simulink model "main"  (R2022a)
settings: Solver=FixedStepDiscrete  StartTime=0.0  StopTime=Inf  FixedStep=(50e-6)-(sim_en*4.995e-5)  RelTol=1e-3  EnableMultiTasking=on
model workspace (MAT data in the model file):
  Param : Simulink.Parameter (value not decoded)
  ac_ok : Simulink.Signal (value not decoded)
  ac_ok_120 : Simulink.Signal (value not decoded)
  bulk_voltage : Simulink.Signal (value not decoded)
  burstduty_integ_max : Simulink.Signal (value not decoded)
  burstduty_integ_min : Simulink.Signal (value not decoded)
  burstduty_ki : Simulink.Signal (value not decoded)
  burstduty_kp : Simulink.Signal (value not decoded)
  calib_ok : Simulink.Signal (value not decoded)
  can_addr1 : Simulink.Signal (value not decoded)
  can_addr2 : Simulink.Signal (value not decoded)
  can_addr3 : Simulink.Signal (value not decoded)
  can_addr4 : Simulink.Signal (value not decoded)
  can_data_rx : Simulink.Signal (value not decoded)
  can_data_tx : Simulink.Signal (value not decoded)
  can_timeout_120 : Simulink.Signal (value not decoded)
  chksum_scircv : Simulink.Signal (value not decoded)
  clllc_en_120 : Simulink.Signal (value not decoded)
  clllc_fault_120 : Simulink.Signal (value not decoded)
  clllc_ok_120 : Simulink.Signal (value not decoded)
  cmpss1h : Simulink.Signal (value not decoded)
  cmpss1l : Simulink.Signal (value not decoded)
  cmpss2h : Simulink.Signal (value not decoded)
  cmpss2l : Simulink.Signal (value not decoded)
  cmpss3h : Simulink.Signal (value not decoded)
  cmpss3l : Simulink.Signal (value not decoded)
  cmpss4h : Simulink.Signal (value not decoded)
  cmpss4l : Simulink.Signal (value not decoded)
  cmpss5h : Simulink.Signal (value not decoded)
  cmpss5l : Simulink.Signal (value not decoded)
  cmpss6h : Simulink.Signal (value not decoded)
  cmpss6l : Simulink.Signal (value not decoded)
  cmpss7h : Simulink.Signal (value not decoded)
  cmpss7l : Simulink.Signal (value not decoded)
  cmpss8h : Simulink.Signal (value not decoded)
  cmpss8l : Simulink.Signal (value not decoded)
  cnt_idle : Simulink.Signal (value not decoded)
  cnt_orps : Simulink.Signal (value not decoded)
  cnt_scircv : Simulink.Signal (value not decoded)
  cnt_scixmt : Simulink.Signal (value not decoded)
  cnt_scixmt_func : Simulink.Signal (value not decoded)
  cnt_temp_mux : Simulink.Signal (value not decoded)
  cnt_vdroop : Simulink.Signal (value not decoded)
  config_ok : Simulink.Signal (value not decoded)
  control_en : Simulink.Signal (value not decoded)
  cp_ready_120 : Simulink.Signal (value not decoded)
  d2d_en : Simulink.Signal (value not decoded)
  dchg_off : Simulink.Signal (value not decoded)
  debug_dacb : Simulink.Signal (value not decoded)
  debug_dacc : Simulink.Signal (value not decoded)
  debug_msg1 : Simulink.Signal (value not decoded)
  debug_msg2 : Simulink.Signal (value not decoded)
  debug_msg3 : Simulink.Signal (value not decoded)
  debug_msg4 : Simulink.Signal (value not decoded)
  debug_msg5 : Simulink.Signal (value not decoded)
  debug_msg6 : Simulink.Signal (value not decoded)
  dir_v2g : Simulink.Signal (value not decoded)
  eoss_llc1 : Simulink.Signal (value not decoded)
  eoss_llc2 : Simulink.Signal (value not decoded)
  eoss_orps : Simulink.Signal (value not decoded)
  fault_ocp : Simulink.Signal (value not decoded)
  fault_otp : Simulink.Signal (value not decoded)
  fault_ovp : Simulink.Signal (value not decoded)
  fut_en : Simulink.Signal (value not decoded)
  fwd_en_120 : Simulink.Signal (value not decoded)
  gain_llc1_sec_idc : Simulink.Signal (value not decoded)
  gain_llc1_temp_sr : Simulink.Signal (value not decoded)
  gain_llc2_sec_idc : Simulink.Signal (value not decoded)
  gain_vbat : Simulink.Signal (value not decoded)
  gain_vbulk : Simulink.Signal (value not decoded)
  gain_vout : Simulink.Signal (value not decoded)
  input_current_phasea : Simulink.Signal (value not decoded)
  input_current_phaseb : Simulink.Signal (value not decoded)
  input_current_phasec : Simulink.Signal (value not decoded)
  input_freq : Simulink.Signal (value not decoded)
  input_power : Simulink.Signal (value not decoded)
  input_voltage_phasea : Simulink.Signal (value not decoded)
  input_voltage_phaseb : Simulink.Signal (value not decoded)
  input_voltage_phasec : Simulink.Signal (value not decoded)
  ishare_arbiter : Simulink.Signal (value not decoded)
  ishare_thresh : Simulink.Signal (value not decoded)
  led_g : Simulink.Signal (value not decoded)
  led_r : Simulink.Signal (value not decoded)
  led_y : Simulink.Signal (value not decoded)
  llc1_burst_integ : Simulink.Signal (value not decoded)
  llc1_burstduty_buffer : Simulink.Signal (value not decoded)
  llc1_pfm_error : Simulink.Signal (value not decoded)
  llc1_pfm_integ : Simulink.Signal (value not decoded)
  llc1_pfm_prop : Simulink.Signal (value not decoded)
  llc1_pri_idc : Simulink.Signal (value not decoded)
  llc1_ps_buffer : Simulink.Signal (value not decoded)
  llc1_pspwm_error : Simulink.Signal (value not decoded)
  llc1_pspwm_integ : Simulink.Signal (value not decoded)
  llc1_pspwm_prop : Simulink.Signal (value not decoded)
  llc1_sec_idc : Simulink.Signal (value not decoded)
  llc1_temp_sr : Simulink.Signal (value not decoded)
  llc1_ts_tbctr_buffer : Simulink.Signal (value not decoded)
  llc2_burst_integ : Simulink.Signal (value not decoded)
  llc2_burstduty_buffer : Simulink.Signal (value not decoded)
  llc2_en : Simulink.Signal (value not decoded)
  llc2_en_buffer : Simulink.Signal (value not decoded)
  llc2_pfm_error : Simulink.Signal (value not decoded)
  llc2_pfm_integ : Simulink.Signal (value not decoded)
  llc2_pfm_prop : Simulink.Signal (value not decoded)
  llc2_pri_idc : Simulink.Signal (value not decoded)
  llc2_ps_buffer : Simulink.Signal (value not decoded)
  llc2_pspwm_error : Simulink.Signal (value not decoded)
  llc2_pspwm_integ : Simulink.Signal (value not decoded)
  llc2_pspwm_prop : Simulink.Signal (value not decoded)
  llc2_sec_idc : Simulink.Signal (value not decoded)
  llc2_temp_sr : Simulink.Signal (value not decoded)
  llc2_ts_tbctr_buffer : Simulink.Signal (value not decoded)
  loop_adcint : Simulink.Signal (value not decoded)
  loop_control : Simulink.Signal (value not decoded)
  loop_idle : Simulink.Signal (value not decoded)
  mid_bulk_voltage : Simulink.Signal (value not decoded)
  mode_120 : Simulink.Signal (value not decoded)
  mode_cc_cv : Simulink.Signal (value not decoded)
  myParam : mpt.Parameter (value not decoded)
  obc_ok_120 : Simulink.Signal (value not decoded)
  offset_llc1_sec_idc : Simulink.Signal (value not decoded)
  offset_llc1_temp_sr : Simulink.Signal (value not decoded)
  offset_llc2_sec_idc : Simulink.Signal (value not decoded)
  offset_vbat : Simulink.Signal (value not decoded)
  offset_vbulk : Simulink.Signal (value not decoded)
  offset_vout : Simulink.Signal (value not decoded)
  openloop_en : Simulink.Signal (value not decoded)
  openloop_fault_en : Simulink.Signal (value not decoded)
  ot_fault_120 : Simulink.Signal (value not decoded)
  pfc_en : Simulink.Signal (value not decoded)
  pfc_en_120 : Simulink.Signal (value not decoded)
  pfc_fw_revision : Simulink.Signal (value not decoded)
  pfc_fw_revision_bootloader : Simulink.Signal (value not decoded)
  pfc_fw_revision_debug : Simulink.Signal (value not decoded)
  pfc_ok : Simulink.Signal (value not decoded)
  pfc_ok_120 : Simulink.Signal (value not decoded)
  pfm_a0 : Simulink.Signal (value not decoded)
  pfm_a1 : Simulink.Signal (value not decoded)
  pfm_integ_max : Simulink.Signal (value not decoded)
  pfm_integ_min : Simulink.Signal (value not decoded)
  pfm_ki : Simulink.Signal (value not decoded)
  pfm_kp : Simulink.Signal (value not decoded)
  pri_fut_en : Simulink.Signal (value not decoded)
  pri_fut_en_buffer : Simulink.Signal (value not decoded)
  pri_halfbridge_en : Simulink.Signal (value not decoded)
  pri_halfbridge_en_buffer : Simulink.Signal (value not decoded)
  pspwm_integ_max : Simulink.Signal (value not decoded)
  pspwm_integ_min : Simulink.Signal (value not decoded)
  pspwm_ki : Simulink.Signal (value not decoded)
  pspwm_kp : Simulink.Signal (value not decoded)
  ref_idclink_max : Simulink.Signal (value not decoded)
  ref_iout : Simulink.Signal (value not decoded)
  ref_iout_calib : Simulink.Signal (value not decoded)
  ref_iout_llc1 : Simulink.Signal (value not decoded)
  ref_iout_llc1_calib : Simulink.Signal (value not decoded)
  ref_iout_llc2 : Simulink.Signal (value not decoded)
  ref_iout_llc2_calib : Simulink.Signal (value not decoded)
  ref_pout : Simulink.Signal (value not decoded)
  ref_ss_llc1 : Simulink.Signal (value not decoded)
  ref_ss_llc2 : Simulink.Signal (value not decoded)
  ref_ss_orps : Simulink.Signal (value not decoded)
  ref_vbat : Simulink.Signal (value not decoded)
  ref_vbat_calib : Simulink.Signal (value not decoded)
  ref_vbulk : Simulink.Signal (value not decoded)
  ref_vbulk_calib : Simulink.Signal (value not decoded)
  ref_vbulk_llc1_calib : Simulink.Signal (value not decoded)
  ref_vbulk_llc2_calib : Simulink.Signal (value not decoded)
  ref_vout : Simulink.Signal (value not decoded)
  ref_vout_calib : Simulink.Signal (value not decoded)
  relay_en : Simulink.Signal (value not decoded)
  reset_flag : Simulink.Signal (value not decoded)
  rev_en_120 : Simulink.Signal (value not decoded)
  runtime_control : Simulink.Signal (value not decoded)
  runtime_idle : Simulink.Signal (value not decoded)
  scircv_buffer : Simulink.Signal (value not decoded)
  scircv_buffer_tmp : Simulink.Signal (value not decoded)
  scircv_buffer_tmp_idx0 : Simulink.Signal (value not decoded)
  scircv_chksum : Simulink.Signal (value not decoded)
  scircv_chksum_ok : Simulink.Signal (value not decoded)
  scircv_parse_ok : Simulink.Signal (value not decoded)
  scixmt_buffer : Simulink.Signal (value not decoded)
  scixmt_chksum : Simulink.Signal (value not decoded)
  scixmt_func : Simulink.Signal (value not decoded)
  scixmt_word0_lsb : Simulink.Signal (value not decoded)
  scixmt_word0_msb : Simulink.Signal (value not decoded)
  scixmt_word1_lsb : Simulink.Signal (value not decoded)
  scixmt_word1_msb : Simulink.Signal (value not decoded)
  scixmt_word2_lsb : Simulink.Signal (value not decoded)
  scixmt_word2_msb : Simulink.Signal (value not decoded)
  scixmt_wr : Simulink.Signal (value not decoded)
  ss_step : Simulink.Signal (value not decoded)
  state_calib : Simulink.Signal (value not decoded)
  state_control : Simulink.Signal (value not decoded)
  state_hkeep : Simulink.Signal (value not decoded)
  status_cmpss : Simulink.Signal (value not decoded)
  status_control : Simulink.Signal (value not decoded)
  status_digin : Simulink.Signal (value not decoded)
  status_digout : Simulink.Signal (value not decoded)
  status_fault : Simulink.Signal (value not decoded)
  status_input : Simulink.Signal (value not decoded)
  status_pfc : Simulink.Signal (value not decoded)
  temp_inlet : Simulink.Signal (value not decoded)
  temp_llc1_fet_hs : Simulink.Signal (value not decoded)
  temp_llc2_fet_hs : Simulink.Signal (value not decoded)
  temp_mux : Simulink.Signal (value not decoded)
  temp_mux_s0 : Simulink.Signal (value not decoded)
  temp_mux_s1 : Simulink.Signal (value not decoded)
  temp_mux_s2 : Simulink.Signal (value not decoded)
  temp_outlet : Simulink.Signal (value not decoded)
  temp_pfc_fet_hsa : Simulink.Signal (value not decoded)
  temp_pfc_fet_hsb : Simulink.Signal (value not decoded)
  temp_pfc_fet_hsc : Simulink.Signal (value not decoded)
  temp_pfc_fet_lsa : Simulink.Signal (value not decoded)
  temp_pfc_fet_lsb : Simulink.Signal (value not decoded)
  temp_pfc_fet_lsc : Simulink.Signal (value not decoded)
  test_mode : Simulink.Signal (value not decoded)
  tfcv_cc : Simulink.Signal (value not decoded)
  tfcv_cc_llc2 : Simulink.Signal (value not decoded)
  tfcv_cv : Simulink.Signal (value not decoded)
  tfcv_sr_en : Simulink.Signal (value not decoded)
  tfv_assert_llc1_pri_idc : Simulink.Signal (value not decoded)
  tfv_assert_llc1_sec_idc : Simulink.Signal (value not decoded)
  tfv_assert_llc1_temp_sr : Simulink.Signal (value not decoded)
  tfv_assert_llc2_pri_idc : Simulink.Signal (value not decoded)
  tfv_assert_llc2_sec_idc : Simulink.Signal (value not decoded)
  tfv_assert_llc2_temp_sr : Simulink.Signal (value not decoded)
  tfv_assert_temp_outlet : Simulink.Signal (value not decoded)
  tfv_assert_vaux_uv : Simulink.Signal (value not decoded)
  tfv_assert_vbat : Simulink.Signal (value not decoded)
  tfv_assert_vbulk : Simulink.Signal (value not decoded)
  tfv_assert_vout : Simulink.Signal (value not decoded)
  tfv_cnt_tz : Simulink.Signal (value not decoded)
  tfv_deassert_llc1_pri_idc : Simulink.Signal (value not decoded)
  tfv_deassert_llc1_sec_idc : Simulink.Signal (value not decoded)
  tfv_deassert_llc1_temp_sr : Simulink.Signal (value not decoded)
  tfv_deassert_llc2_pri_idc : Simulink.Signal (value not decoded)
  tfv_deassert_llc2_sec_idc : Simulink.Signal (value not decoded)
  tfv_deassert_llc2_temp_sr : Simulink.Signal (value not decoded)
  tfv_deassert_temp_outlet : Simulink.Signal (value not decoded)
  tfv_deassert_vaux_uv : Simulink.Signal (value not decoded)
  tfv_deassert_vbat : Simulink.Signal (value not decoded)
  tfv_deassert_vbulk : Simulink.Signal (value not decoded)
  tfv_deassert_vout : Simulink.Signal (value not decoded)
  tfv_llc1_pri_idc : Simulink.Signal (value not decoded)
  tfv_llc1_sec_idc : Simulink.Signal (value not decoded)
  tfv_llc1_temp_sr : Simulink.Signal (value not decoded)
  tfv_llc2_pri_idc : Simulink.Signal (value not decoded)
  tfv_llc2_sec_idc : Simulink.Signal (value not decoded)
  tfv_llc2_temp_sr : Simulink.Signal (value not decoded)
  tfv_temp_outlet : Simulink.Signal (value not decoded)
  tfv_vaux_uv : Simulink.Signal (value not decoded)
  tfv_vbat : Simulink.Signal (value not decoded)
  tfv_vbulk : Simulink.Signal (value not decoded)
  tfv_vout : Simulink.Signal (value not decoded)
  timer_1ms : Simulink.Signal (value not decoded)
  tz : Simulink.Signal (value not decoded)
  valve_en : Simulink.Signal (value not decoded)
  vaux : Simulink.Signal (value not decoded)
  vbat : Simulink.Signal (value not decoded)
  vbulk : Simulink.Signal (value not decoded)
  vout : Simulink.Signal (value not decoded)
undefined symbols (not defined in the file or in its folder): CAN_O_INT, CANA_BASE, Down, GPTRIP1SEL, GPTRIP2SEL, TZ1, TZ2, Up
libraries: hdlsllib x159, simulink x94, c2802xlib x32, c2837xDlib x19, c2807xlib x16, c280xlib x13, canmsglib x8, idelinklib_common x2, c2000lib x1, c281xlib x1
(part 18 of 20)

== system main/Task_Manager/Tmr_20mS/codegen/Task_20mS/Tx_Handler/Run Tx Routine/TxReadRequest/Tx TxDeb Dat2 147 ==
  Action Port : ActionPort  ActionPortLabel=case [ 210 ]:
  CAN Pack1 : canmsglib/CAN Pack  MsgList=(none)  MsgName=CAN Msg  MsgIDType=Standard (11-bit identifier)  MsgIdentifier=0x147  MsgLength=8  Remote=off  ApplyMinMax=off  BusOutput=off  SignalInfo={}
      settings: SourceProductBaseCode=XP,ME,VN  DataFormat=raw data
  Constant4 : Constant  Value=0  OutDataTypeStr=uint8
  Data Store Read1 : DataStoreRead  DataStoreName=u16Debug3  IndexOptions=Index vector (dialog)  Indices=1  OutputSizes=1
  Data Store Read2 : DataStoreRead  DataStoreName=u16Debug4  IndexOptions=Index vector (dialog)  Indices=1  OutputSizes=1
  Data Store Read3 : DataStoreRead  DataStoreName=u16Debug5  IndexOptions=Index vector (dialog)  Indices=1  OutputSizes=1
  Vector Concatenate : Concatenate  NumInputs=8
  eCAN Transmit : c280xlib/eCAN Transmit  chipFamily=C280x  useModule=eCAN_A  mailboxNo=8  messageID=hex2dec('0147')  messageType=Standard (11-bit identifier)  enableBlockingMode=off  postInterrupt=off  interruptLine=0
      settings: SourceProductBaseCode=TIC2000
  u16 Data to Bytes : Subsystem
  u16 Data to Bytes1 : Subsystem
  u16 Data to Bytes2 : Subsystem
  wires:
  u16 Data to Bytes1/2(u8Msb) -> Vector Concatenate/6
  u16 Data to Bytes2/2(u8Msb) -> Vector Concatenate/4
  u16 Data to Bytes1/1(u8Lsb) -> Vector Concatenate/5
  Data Store Read1/1 -> u16 Data to Bytes/1(u16 Data)
  Data Store Read3/1 -> u16 Data to Bytes1/1(u16 Data)
  Vector Concatenate/1 -> CAN Pack1/1
  u16 Data to Bytes/1(u8Lsb) -> Vector Concatenate/1
  CAN Pack1/1 -> eCAN Transmit/1
  Data Store Read2/1 -> u16 Data to Bytes2/1(u16 Data)
  u16 Data to Bytes/2(u8Msb) -> Vector Concatenate/2
  Constant4/1 -> Vector Concatenate/8, Vector Concatenate/7
  u16 Data to Bytes2/1(u8Lsb) -> Vector Concatenate/3

== system main/Task_Manager/Tmr_20mS/codegen/Task_20mS/Tx_Handler/Run Tx Routine/TxStatusData/Tx Sec Status ID120 ==
  Action Port : ActionPort  ActionPortLabel=case [ 0 ]:
  CAN Pack1 : canmsglib/CAN Pack  MsgList=(none)  MsgName=CAN Msg  MsgIDType=Standard (11-bit identifier)  MsgIdentifier=0x120  MsgLength=8  Remote=off  ApplyMinMax=off  BusOutput=off  SignalInfo={}
      settings: SourceProductBaseCode=XP,ME,VN  DataFormat=raw data
  Constant1 : Constant  Value=0.1  OutDataTypeStr=single
  Constant3 : Constant  Value=0.01  OutDataTypeStr=single
  Constant4 : Constant  Value=0.1  OutDataTypeStr=single
  Data Store Read1 : DataStoreRead  DataStoreName=sSecStatus  IndexOptions=Index vector (dialog)  Indices=1  OutputSizes=1
  Data Store Read2 : DataStoreRead  DataStoreName=f32Vout  IndexOptions=Index vector (dialog)  Indices=1  OutputSizes=1
  Data Store Read3 : DataStoreRead  DataStoreName=b00_DebugEnabled  IndexOptions=Index vector (dialog)  Indices=1  OutputSizes=1
  Data Store Read4 : DataStoreRead  DataStoreName=f32Iout  IndexOptions=Index vector (dialog)  Indices=1  OutputSizes=1
  Data Store Read5 : DataStoreRead  DataStoreName=f32Vbulk  IndexOptions=Index vector (dialog)  Indices=1  OutputSizes=1
  Float Data to Bytes : Subsystem
  Float Data to Bytes1 : Subsystem
  Float Data to Bytes2 : Subsystem
  If1 : If  IfExpression=u1 == 1
  TxReadRequest : Subsystem  TreatAsAtomicUnit=on
  Vector Concatenate : Concatenate  NumInputs=8
  eCAN Transmit : c280xlib/eCAN Transmit  chipFamily=C280x  useModule=eCAN_A  mailboxNo=0  messageID=hex2dec('0120')  messageType=Standard (11-bit identifier)  enableBlockingMode=off  postInterrupt=off  interruptLine=0
      settings: SourceProductBaseCode=TIC2000
  u16 Data to Bytes : Subsystem
  wires:
  CAN Pack1/1 -> eCAN Transmit/1
  Data Store Read3/1 -> If1/1
  If1/1 -> TxReadRequest/Action
  Data Store Read1/1 -> u16 Data to Bytes/1(u16 Data)
  u16 Data to Bytes/1(u8Lsb) -> Vector Concatenate/1
  u16 Data to Bytes/2(u8Msb) -> Vector Concatenate/2
  Vector Concatenate/1 -> CAN Pack1/1
  Constant1/1 -> Float Data to Bytes/2(Resol.)
  Data Store Read2/1 -> Float Data to Bytes/1(Float Data)
  Float Data to Bytes/1(u8Lsb) -> Vector Concatenate/3
  Float Data to Bytes/2(u8Msb) -> Vector Concatenate/4
  Data Store Read4/1 -> Float Data to Bytes1/1(Float Data)
  Constant3/1 -> Float Data to Bytes1/2(Resol.)
  Constant4/1 -> Float Data to Bytes2/2(Resol.)
  Data Store Read5/1 -> Float Data to Bytes2/1(Float Data)
  Float Data to Bytes1/1(u8Lsb) -> Vector Concatenate/5
  Float Data to Bytes1/2(u8Msb) -> Vector Concatenate/6
  Float Data to Bytes2/1(u8Lsb) -> Vector Concatenate/7
  Float Data to Bytes2/2(u8Msb) -> Vector Concatenate/8

== system main/Task_Manager/Tmr_20mS/codegen/Task_20mS/Tx_Handler/Run Tx Routine/TxStatusData/Tx Sec1 ID140 ==
  Action Port : ActionPort  ActionPortLabel=case [ 1 ]:
  CAN Pack1 : canmsglib/CAN Pack  MsgList=(none)  MsgName=CAN Msg  MsgIDType=Standard (11-bit identifier)  MsgIdentifier=0x140  MsgLength=8  Remote=off  ApplyMinMax=off  BusOutput=off  SignalInfo={}
      settings: SourceProductBaseCode=XP,ME,VN  DataFormat=raw data
  Constant1 : Constant  Value=2  OutDataTypeStr=uint8
  Constant4 : Constant  Value=0.01  OutDataTypeStr=single
  Data Store Read1 : DataStoreRead  DataStoreName=sSecFault  IndexOptions=Index vector (dialog)  Indices=1  OutputSizes=1
  Data Store Read2 : DataStoreRead  DataStoreName=u16Reserved1  IndexOptions=Index vector (dialog)  Indices=1  OutputSizes=1
  Data Store Read3 : DataStoreRead  DataStoreName=u16Reserved2  IndexOptions=Index vector (dialog)  Indices=1  OutputSizes=1
  Data Store Read5 : DataStoreRead  DataStoreName=f32PriCurrRev  IndexOptions=Index vector (dialog)  Indices=1  OutputSizes=1
  Data Store Write1 : DataStoreWrite  DataStoreName=u8CanTxIndex  IndexOptions=Index vector (dialog)  Indices=1  OutputSizes=1
  Float Data to Bytes2 : Subsystem
  Vector Concatenate : Concatenate  NumInputs=8
  eCAN Transmit : c280xlib/eCAN Transmit  chipFamily=C280x  useModule=eCAN_A  mailboxNo=1  messageID=hex2dec('0140')  messageType=Standard (11-bit identifier)  enableBlockingMode=off  postInterrupt=off  interruptLine=0
      settings: SourceProductBaseCode=TIC2000
  u16 Data to Bytes : Subsystem
  u16 Data to Bytes1 : Subsystem
  u16 Data to Bytes2 : Subsystem
  wires:
  Constant1/1 -> Data Store Write1/1
  Data Store Read2/1 -> u16 Data to Bytes2/1(u16 Data)
  CAN Pack1/1 -> eCAN Transmit/1
  u16 Data to Bytes2/1(u8Lsb) -> Vector Concatenate/3
  u16 Data to Bytes/1(u8Lsb) -> Vector Concatenate/1
  u16 Data to Bytes/2(u8Msb) -> Vector Concatenate/2
  Float Data to Bytes2/2(u8Msb) -> Vector Concatenate/8
  Constant4/1 -> Float Data to Bytes2/2(Resol.)
  Float Data to Bytes2/1(u8Lsb) -> Vector Concatenate/7
  Data Store Read5/1 -> Float Data to Bytes2/1(Float Data)
  u16 Data to Bytes2/2(u8Msb) -> Vector Concatenate/4
  Data Store Read1/1 -> u16 Data to Bytes/1(u16 Data)
  u16 Data to Bytes1/1(u8Lsb) -> Vector Concatenate/5
  Vector Concatenate/1 -> CAN Pack1/1
  u16 Data to Bytes1/2(u8Msb) -> Vector Concatenate/6
  Data Store Read3/1 -> u16 Data to Bytes1/1(u16 Data)

== system main/Task_Manager/Tmr_20mS/codegen/Task_20mS/Tx_Handler/Run Tx Routine/TxStatusData/Tx Sec2 ID141 ==
  Action Port : ActionPort  ActionPortLabel=case [ 2 ]:
  CAN Pack1 : canmsglib/CAN Pack  MsgList=(none)  MsgName=CAN Msg  MsgIDType=Standard (11-bit identifier)  MsgIdentifier=0x141  MsgLength=8  Remote=off  ApplyMinMax=off  BusOutput=off  SignalInfo={}
      settings: SourceProductBaseCode=XP,ME,VN  DataFormat=raw data
  Constant1 : Constant  Value=3  OutDataTypeStr=uint8
  Constant{2..5} (4 alike) : Constant  Value=0.01  OutDataTypeStr=single
  Data Store Read1 : DataStoreRead  DataStoreName=f32Iout1  IndexOptions=Index vector (dialog)  Indices=1  OutputSizes=1
  Data Store Read2 : DataStoreRead  DataStoreName=f32Iout2  IndexOptions=Index vector (dialog)  Indices=1  OutputSizes=1
  Data Store Read4 : DataStoreRead  DataStoreName=f32PriCurrRev1  IndexOptions=Index vector (dialog)  Indices=1  OutputSizes=1
  Data Store Read5 : DataStoreRead  DataStoreName=f32PriCurrRev2  IndexOptions=Index vector (dialog)  Indices=1  OutputSizes=1
  Data Store Write1 : DataStoreWrite  DataStoreName=u8CanTxIndex  IndexOptions=Index vector (dialog)  Indices=1  OutputSizes=1
  Float Data to Bytes : Subsystem
  Float Data to Bytes1 : Subsystem
  Float Data to Bytes2 : Subsystem
  Float Data to Bytes3 : Subsystem
  Vector Concatenate : Concatenate  NumInputs=8
  eCAN Transmit : c280xlib/eCAN Transmit  chipFamily=C280x  useModule=eCAN_A  mailboxNo=2  messageID=hex2dec('0141')  messageType=Standard (11-bit identifier)  enableBlockingMode=off  postInterrupt=off  interruptLine=0
      settings: SourceProductBaseCode=TIC2000
  wires:
  Constant1/1 -> Data Store Write1/1
  Data Store Read4/1 -> Float Data to Bytes1/1(Float Data)
  Data Store Read2/1 -> Float Data to Bytes/1(Float Data)
  Constant2/1 -> Float Data to Bytes/2(Resol.)
  CAN Pack1/1 -> eCAN Transmit/1
  Float Data to Bytes/1(u8Lsb) -> Vector Concatenate/3
  Float Data to Bytes3/1(u8Lsb) -> Vector Concatenate/1
  Float Data to Bytes3/2(u8Msb) -> Vector Concatenate/2
  Float Data to Bytes2/2(u8Msb) -> Vector Concatenate/8
  Constant4/1 -> Float Data to Bytes2/2(Resol.)
  Float Data to Bytes2/1(u8Lsb) -> Vector Concatenate/7
  Data Store Read5/1 -> Float Data to Bytes2/1(Float Data)
  Float Data to Bytes/2(u8Msb) -> Vector Concatenate/4
  Data Store Read1/1 -> Float Data to Bytes3/1(Float Data)
  Float Data to Bytes1/1(u8Lsb) -> Vector Concatenate/5
  Vector Concatenate/1 -> CAN Pack1/1
  Constant3/1 -> Float Data to Bytes1/2(Resol.)
  Float Data to Bytes1/2(u8Msb) -> Vector Concatenate/6
  Constant5/1 -> Float Data to Bytes3/2(Resol.)

== system main/Task_Manager/Tmr_20mS/codegen/Task_20mS/Tx_Handler/Run Tx Routine/TxStatusData/Tx Sec3 ID142 ==
  Action Port : ActionPort  ActionPortLabel=case [ 3 ]:
  CAN Pack1 : canmsglib/CAN Pack  MsgList=(none)  MsgName=CAN Msg  MsgIDType=Standard (11-bit identifier)  MsgIdentifier=0x142  MsgLength=8  Remote=off  ApplyMinMax=off  BusOutput=off  SignalInfo={}
      settings: SourceProductBaseCode=XP,ME,VN  DataFormat=raw data
  Constant1 : Constant  Value=4  OutDataTypeStr=uint8
  Constant3 : Constant  Value=0.1  OutDataTypeStr=single
  Constant4 : Constant  Value=0.1  OutDataTypeStr=single
  Data Store Read1 : DataStoreRead  DataStoreName=u8TclllcS1  IndexOptions=Index vector (dialog)  Indices=1  OutputSizes=1
  Data Store Read2 : DataStoreRead  DataStoreName=u8TclllcS3  IndexOptions=Index vector (dialog)  Indices=1  OutputSizes=1
  Data Store Read3 : DataStoreRead  DataStoreName=u8TclllcS2  IndexOptions=Index vector (dialog)  Indices=1  OutputSizes=1
  Data Store Read4 : DataStoreRead  DataStoreName=f32IshareErr  IndexOptions=Index vector (dialog)  Indices=1  OutputSizes=1
  Data Store Read5 : DataStoreRead  DataStoreName=f32IshareAdj  IndexOptions=Index vector (dialog)  Indices=1  OutputSizes=1
  Data Store Read6 : DataStoreRead  DataStoreName=u8TclllcS4  IndexOptions=Index vector (dialog)  Indices=1  OutputSizes=1
  Data Store Write1 : DataStoreWrite  DataStoreName=u8CanTxIndex  IndexOptions=Index vector (dialog)  Indices=1  OutputSizes=1
  Float Data to Signed Bytes : Subsystem
  Float Data to Signed Bytes1 : Subsystem
  Vector Concatenate : Concatenate  NumInputs=8
  eCAN Transmit : c280xlib/eCAN Transmit  chipFamily=C280x  useModule=eCAN_A  mailboxNo=3  messageID=hex2dec('0142')  messageType=Standard (11-bit identifier)  enableBlockingMode=off  postInterrupt=off  interruptLine=0
      settings: SourceProductBaseCode=TIC2000
  wires:
  Constant1/1 -> Data Store Write1/1
  Data Store Read4/1 -> Float Data to Signed Bytes/1(Float Data)
  CAN Pack1/1 -> eCAN Transmit/1
  Data Store Read1/1 -> Vector Concatenate/1
  Data Store Read3/1 -> Vector Concatenate/2
  Float Data to Signed Bytes1/2(u8Msb) -> Vector Concatenate/8
  Constant4/1 -> Float Data to Signed Bytes1/2(Resol.)
  Float Data to Signed Bytes1/1(u8Lsb) -> Vector Concatenate/7
  Data Store Read5/1 -> Float Data to Signed Bytes1/1(Float Data)
  Float Data to Signed Bytes/1(u8Lsb) -> Vector Concatenate/5
  Vector Concatenate/1 -> CAN Pack1/1
  Constant3/1 -> Float Data to Signed Bytes/2(Resol.)
  Float Data to Signed Bytes/2(u8Msb) -> Vector Concatenate/6
  Data Store Read6/1 -> Vector Concatenate/4
  Data Store Read2/1 -> Vector Concatenate/3

== system main/Task_Manager/Tmr_20mS/codegen/Task_20mS/Tx_Handler/Run Tx Routine/TxStatusData/Tx Sec4 ID143 ==
  Action Port : ActionPort  ActionPortLabel=case [ 4 ]:
  Bit Shift : hdlsllib/Logic and Bit Operations/Bit Shift  mode=Shift Left Logical  N=4
  Bitwise AND : simulink/Logic and Bit Operations/Bitwise Operator  logicop=AND  UseBitMask=on  BitMask=bin2dec('00001111')  BitMaskRealWorld=Stored Integer
  Bitwise AND1 : simulink/Logic and Bit Operations/Bitwise Operator  logicop=AND  UseBitMask=on  BitMask=hex2dec('0F')  BitMaskRealWorld=Stored Integer
  Bitwise AND2 : simulink/Logic and Bit Operations/Bitwise Operator  logicop=OR  UseBitMask=off  NumInputPorts=2  BitMask=bin2dec('00001111')  BitMaskRealWorld=Stored Integer
  CAN Pack1 : canmsglib/CAN Pack  MsgList=(none)  MsgName=CAN Msg  MsgIDType=Standard (11-bit identifier)  MsgIdentifier=0x143  MsgLength=8  Remote=off  ApplyMinMax=off  BusOutput=off  SignalInfo={}
      settings: SourceProductBaseCode=XP,ME,VN  DataFormat=raw data
  Constant1 : Constant  Value=0  OutDataTypeStr=uint8
  Constant3 : Constant  Value=0.1  OutDataTypeStr=single
  Constant4 : Constant  Value=0.1  OutDataTypeStr=single
  Data Store Read1 : DataStoreRead  DataStoreName=sSecCtrlState  IndexOptions=Index vector (dialog)  Indices=1  OutputSizes=1
  Data Store Read2 : DataStoreRead  DataStoreName=u8PhaseShift1  IndexOptions=Index vector (dialog)  Indices=1  OutputSizes=1
  Data Store Read3 : DataStoreRead  DataStoreName=u8PhaseShift2  IndexOptions=Index vector (dialog)  Indices=1  OutputSizes=1
  Data Store Read4 : DataStoreRead  DataStoreName=f32Period1  IndexOptions=Index vector (dialog)  Indices=1  OutputSizes=1
  Data Store Read5 : DataStoreRead  DataStoreName=f32Period2  IndexOptions=Index vector (dialog)  Indices=1  OutputSizes=1
  Data Store Read6 : DataStoreRead  DataStoreName=u8BurstDty1  IndexOptions=Index vector (dialog)  Indices=1  OutputSizes=1
  Data Store Read7 : DataStoreRead  DataStoreName=u8BurstDty2  IndexOptions=Index vector (dialog)  Indices=1  OutputSizes=1
  Data Store Read8 : DataStoreRead  DataStoreName=u8BurstDty1  IndexOptions=Index vector (dialog)  Indices=1  OutputSizes=1
  Data Store Write1 : DataStoreWrite  DataStoreName=u8CanTxIndex  IndexOptions=Index vector (dialog)  Indices=1  OutputSizes=1
  Float Data to Bytes1 : Subsystem
  Float Data to Bytes2 : Subsystem
  Vector Concatenate : Concatenate  NumInputs=8
  eCAN Transmit : c280xlib/eCAN Transmit  chipFamily=C280x  useModule=eCAN_A  mailboxNo=4  messageID=hex2dec('0143')  messageType=Standard (11-bit identifier)  enableBlockingMode=off  postInterrupt=off  interruptLine=0
      settings: SourceProductBaseCode=TIC2000
  wires:
  Constant1/1 -> Data Store Write1/1
  Data Store Read4/1 -> Float Data to Bytes1/1(Float Data)
  CAN Pack1/1 -> eCAN Transmit/1
  Data Store Read1/1 -> Vector Concatenate/1
  Float Data to Bytes2/2(u8Msb) -> Vector Concatenate/8
  Constant4/1 -> Float Data to Bytes2/2(Resol.)
  Float Data to Bytes2/1(u8Lsb) -> Vector Concatenate/7
  Data Store Read5/1 -> Float Data to Bytes2/1(Float Data)
  Float Data to Bytes1/1(u8Lsb) -> Vector Concatenate/5
  Vector Concatenate/1 -> CAN Pack1/1
  Constant3/1 -> Float Data to Bytes1/2(Resol.)
  Float Data to Bytes1/2(u8Msb) -> Vector Concatenate/6
  Data Store Read2/1 -> Vector Concatenate/3
  Data Store Read3/1 -> Vector Concatenate/4
  Bitwise AND/1 -> Bitwise AND2/1
  Bitwise AND1/1 -> Bit Shift/1
  Bit Shift/1 -> Bitwise AND2/2
  Data Store Read7/1 -> Bitwise AND1/1
  Data Store Read6/1 -> Bitwise AND/1
  Data Store Read8/1 -> Vector Concatenate/2

== system main/Task_Manager/idle/idle_task/comm_npc/comm_npc/COMM_NPC.parseScircv/For Iterator Subsystem/header_found_before_bit13/copy_to_scixmt_buffer ==
  function : TriggerPort  TriggerType=function-call  VariantControl=Variant
  For Iterator Subsystem1 : Subsystem  TreatAsAtomicUnit=on

== system main/Task_Manager/idle/idle_task/comm_npc/comm_npc/COMM_NPC.parseScircv/For Iterator Subsystem/header_found_before_bit13/scircv_parse_ok ==
  function : TriggerPort  TriggerType=function-call  VariantControl=Variant
  Constant : Constant  OutDataTypeStr=boolean
  Out1 : Outport
  wires:
  Constant/1 -> Out1/1

== system main/Task_Manager/idle/idle_task/comm_npc/comm_npc/COMM_NPC.parseScircv/For Iterator Subsystem/header_found_before_bit13/update_scircv_buffer_tmp_idx0 ==
  Inport : Inport
  function : TriggerPort  TriggerType=function-call  VariantControl=Variant
  Data Store Write : DataStoreWrite  DataStoreName=scircv_buffer_tmp_idx0  IndexOptions=Index vector (dialog)  Indices=1  OutputSizes=1
  wires:
  Inport/1 -> Data Store Write/1

== system main/Task_Manager/Tmr_20mS/codegen/Task_20mS/Rx_Handler/ProcessMB12/Debug_Cmd/Debug En//Dis/Debug_Dis ==
  Action Port : ActionPort  ActionPortLabel=elseif(u1 ==hex2dec('55'))
  Constant : Constant  Value=0  OutDataTypeStr=boolean
  Data Store Write1 : DataStoreWrite  DataStoreName=b00_DebugEnabled  IndexOptions=Index vector (dialog)  Indices=1  OutputSizes=1
  wires:
  Constant/1 -> Data Store Write1/1

== system main/Task_Manager/Tmr_20mS/codegen/Task_20mS/Rx_Handler/ProcessMB12/Debug_Cmd/Debug En//Dis/Debug_En ==
  Action Port : ActionPort  ActionPortLabel=if(u1 == hex2dec('AA'))
  Constant : Constant  OutDataTypeStr=boolean
  Data Store Write1 : DataStoreWrite  DataStoreName=b00_DebugEnabled  IndexOptions=Index vector (dialog)  Indices=1  OutputSizes=1
  wires:
  Constant/1 -> Data Store Write1/1

== system main/Task_Manager/Tmr_20mS/codegen/Task_20mS/Rx_Handler/ProcessMB12/Debug_Cmd/Open Loop En Dis/Disable Open Loop ==
  Action Port : ActionPort  ActionPortLabel=elseif(u1 ==hex2dec('44'))
  Constant : Constant  Value=0  OutDataTypeStr=uint8
  Data Store Write1 : DataStoreWrite  DataStoreName=u8OpenLoopEn1  IndexOptions=Index vector (dialog)  Indices=1  OutputSizes=1
  Data Store Write2 : DataStoreWrite  DataStoreName=u8OpenLoopEn2  IndexOptions=Index vector (dialog)  Indices=1  OutputSizes=1
  wires:
  Constant/1 -> Data Store Write2/1, Data Store Write1/1

== system main/Task_Manager/Tmr_20mS/codegen/Task_20mS/Rx_Handler/ProcessMB12/Debug_Cmd/Open Loop En Dis/Enable Open Loop ==
  Action Port : ActionPort  ActionPortLabel=if(u1 == hex2dec('BB'))
  CLLLC1 ON : Subsystem  TreatAsAtomicUnit=on
  CLLLC2 ON : Subsystem  TreatAsAtomicUnit=on
  Constant3 : Constant  Value=[3:3]
  Data Store Read1 : DataStoreRead  DataStoreName=u8CanDataRx12  IndexOptions=Index vector (dialog)  Indices=1  OutputSizes=1
  If1 : If  IfExpression=u1 == 1  ElseIfExpressions=u1 == 2
  Selector3 : Selector  IndexMode=Zero-based  InputPortWidth=8  IndexOptions=Index vector (port)  Indices=[1 3]  OutputSizes=1
  wires:
  Data Store Read1/1 -> Selector3/1
  Selector3/1 -> If1/1
  Constant3/1 -> Selector3/2
  If1/1 -> CLLLC1 ON/Action
  If1/2 -> CLLLC2 ON/Action

== system main/Task_Manager/Tmr_20mS/codegen/Task_20mS/Tx_Handler/Run Tx Routine/TxReadRequest/Tx TxDeb Dat1 146/u16 Data to Bytes ==
  u16 Data : Inport
  Bit Shift : hdlsllib/Logic and Bit Operations/Bit Shift  mode=Shift Right Logical  N=8
  Bitwise AND : simulink/Logic and Bit Operations/Bitwise Operator  logicop=AND  UseBitMask=on  BitMask=bin2dec('0000000011111111')  BitMaskRealWorld=Stored Integer
  Bitwise AND1 : simulink/Logic and Bit Operations/Bitwise Operator  logicop=AND  UseBitMask=on  BitMask=hex2dec('FF00')  BitMaskRealWorld=Stored Integer
  Data Type Conversion : DataTypeConversion  OutDataTypeStr=uint8  SaturateOnIntegerOverflow=off  RndMeth=Floor
  Data Type Conversion1 : DataTypeConversion  OutDataTypeStr=uint8  SaturateOnIntegerOverflow=off  RndMeth=Floor
  u8Lsb : Outport
  u8Msb : Outport  Port=2
  wires:
  u16 Data/1 -> Bitwise AND1/1, Bitwise AND/1
  Bit Shift/1 -> Data Type Conversion1/1
  Bitwise AND/1 -> Data Type Conversion/1
  Data Type Conversion1/1 -> u8Msb/1
  Bitwise AND1/1 -> Bit Shift/1
  Data Type Conversion/1 -> u8Lsb/1

== system main/Task_Manager/Tmr_20mS/codegen/Task_20mS/Tx_Handler/Run Tx Routine/TxReadRequest/Tx TxDeb Dat1 146/u16 Data to Bytes1 ==
  u16 Data : Inport
  Bit Shift : hdlsllib/Logic and Bit Operations/Bit Shift  mode=Shift Right Logical  N=8
  Bitwise AND : simulink/Logic and Bit Operations/Bitwise Operator  logicop=AND  UseBitMask=on  BitMask=bin2dec('0000000011111111')  BitMaskRealWorld=Stored Integer
  Bitwise AND1 : simulink/Logic and Bit Operations/Bitwise Operator  logicop=AND  UseBitMask=on  BitMask=hex2dec('FF00')  BitMaskRealWorld=Stored Integer
  Data Type Conversion : DataTypeConversion  OutDataTypeStr=uint8  SaturateOnIntegerOverflow=off  RndMeth=Floor
  Data Type Conversion1 : DataTypeConversion  OutDataTypeStr=uint8  SaturateOnIntegerOverflow=off  RndMeth=Floor
  u8Lsb : Outport
  u8Msb : Outport  Port=2
  wires:
  Data Type Conversion/1 -> u8Lsb/1
  Bitwise AND1/1 -> Bit Shift/1
  Data Type Conversion1/1 -> u8Msb/1
  Bitwise AND/1 -> Data Type Conversion/1
  Bit Shift/1 -> Data Type Conversion1/1
  u16 Data/1 -> Bitwise AND/1, Bitwise AND1/1

== system main/Task_Manager/Tmr_20mS/codegen/Task_20mS/Tx_Handler/Run Tx Routine/TxReadRequest/Tx TxDeb Dat1 146/u16 Data to Bytes2 ==
  u16 Data : Inport
  Bit Shift : hdlsllib/Logic and Bit Operations/Bit Shift  mode=Shift Right Logical  N=8
  Bitwise AND : simulink/Logic and Bit Operations/Bitwise Operator  logicop=AND  UseBitMask=on  BitMask=bin2dec('0000000011111111')  BitMaskRealWorld=Stored Integer
  Bitwise AND1 : simulink/Logic and Bit Operations/Bitwise Operator  logicop=AND  UseBitMask=on  BitMask=hex2dec('FF00')  BitMaskRealWorld=Stored Integer
  Data Type Conversion : DataTypeConversion  OutDataTypeStr=uint8  SaturateOnIntegerOverflow=off  RndMeth=Floor
  Data Type Conversion1 : DataTypeConversion  OutDataTypeStr=uint8  SaturateOnIntegerOverflow=off  RndMeth=Floor
  u8Lsb : Outport
  u8Msb : Outport  Port=2
  wires:
  u16 Data/1 -> Bitwise AND1/1, Bitwise AND/1
  Bit Shift/1 -> Data Type Conversion1/1
  Bitwise AND/1 -> Data Type Conversion/1
  Data Type Conversion1/1 -> u8Msb/1
  Bitwise AND1/1 -> Bit Shift/1
  Data Type Conversion/1 -> u8Lsb/1

== system main/Task_Manager/Tmr_20mS/codegen/Task_20mS/Tx_Handler/Run Tx Routine/TxReadRequest/Tx TxDeb Dat2 147/u16 Data to Bytes ==
  u16 Data : Inport
  Bit Shift : hdlsllib/Logic and Bit Operations/Bit Shift  mode=Shift Right Logical  N=8
  Bitwise AND : simulink/Logic and Bit Operations/Bitwise Operator  logicop=AND  UseBitMask=on  BitMask=bin2dec('0000000011111111')  BitMaskRealWorld=Stored Integer
  Bitwise AND1 : simulink/Logic and Bit Operations/Bitwise Operator  logicop=AND  UseBitMask=on  BitMask=hex2dec('FF00')  BitMaskRealWorld=Stored Integer
  Data Type Conversion : DataTypeConversion  OutDataTypeStr=uint8  SaturateOnIntegerOverflow=off  RndMeth=Floor
  Data Type Conversion1 : DataTypeConversion  OutDataTypeStr=uint8  SaturateOnIntegerOverflow=off  RndMeth=Floor
  u8Lsb : Outport
  u8Msb : Outport  Port=2
  wires:
  u16 Data/1 -> Bitwise AND1/1, Bitwise AND/1
  Bit Shift/1 -> Data Type Conversion1/1
  Bitwise AND/1 -> Data Type Conversion/1
  Data Type Conversion1/1 -> u8Msb/1
  Bitwise AND1/1 -> Bit Shift/1
  Data Type Conversion/1 -> u8Lsb/1

== system main/Task_Manager/Tmr_20mS/codegen/Task_20mS/Tx_Handler/Run Tx Routine/TxReadRequest/Tx TxDeb Dat2 147/u16 Data to Bytes1 ==
  u16 Data : Inport
  Bit Shift : hdlsllib/Logic and Bit Operations/Bit Shift  mode=Shift Right Logical  N=8
  Bitwise AND : simulink/Logic and Bit Operations/Bitwise Operator  logicop=AND  UseBitMask=on  BitMask=bin2dec('0000000011111111')  BitMaskRealWorld=Stored Integer
  Bitwise AND1 : simulink/Logic and Bit Operations/Bitwise Operator  logicop=AND  UseBitMask=on  BitMask=hex2dec('FF00')  BitMaskRealWorld=Stored Integer
  Data Type Conversion : DataTypeConversion  OutDataTypeStr=uint8  SaturateOnIntegerOverflow=off  RndMeth=Floor
  Data Type Conversion1 : DataTypeConversion  OutDataTypeStr=uint8  SaturateOnIntegerOverflow=off  RndMeth=Floor
  u8Lsb : Outport
  u8Msb : Outport  Port=2
  wires:
  Data Type Conversion/1 -> u8Lsb/1
  Bitwise AND1/1 -> Bit Shift/1
  Data Type Conversion1/1 -> u8Msb/1
  Bitwise AND/1 -> Data Type Conversion/1
  Bit Shift/1 -> Data Type Conversion1/1
  u16 Data/1 -> Bitwise AND/1, Bitwise AND1/1

== system main/Task_Manager/Tmr_20mS/codegen/Task_20mS/Tx_Handler/Run Tx Routine/TxReadRequest/Tx TxDeb Dat2 147/u16 Data to Bytes2 ==
  u16 Data : Inport
  Bit Shift : hdlsllib/Logic and Bit Operations/Bit Shift  mode=Shift Right Logical  N=8
  Bitwise AND : simulink/Logic and Bit Operations/Bitwise Operator  logicop=AND  UseBitMask=on  BitMask=bin2dec('0000000011111111')  BitMaskRealWorld=Stored Integer
  Bitwise AND1 : simulink/Logic and Bit Operations/Bitwise Operator  logicop=AND  UseBitMask=on  BitMask=hex2dec('FF00')  BitMaskRealWorld=Stored Integer
  Data Type Conversion : DataTypeConversion  OutDataTypeStr=uint8  SaturateOnIntegerOverflow=off  RndMeth=Floor
  Data Type Conversion1 : DataTypeConversion  OutDataTypeStr=uint8  SaturateOnIntegerOverflow=off  RndMeth=Floor
  u8Lsb : Outport
  u8Msb : Outport  Port=2
  wires:
  u16 Data/1 -> Bitwise AND1/1, Bitwise AND/1
  Bit Shift/1 -> Data Type Conversion1/1
  Bitwise AND/1 -> Data Type Conversion/1
  Data Type Conversion1/1 -> u8Msb/1
  Bitwise AND1/1 -> Bit Shift/1
  Data Type Conversion/1 -> u8Lsb/1

== system main/Task_Manager/Tmr_20mS/codegen/Task_20mS/Tx_Handler/Run Tx Routine/TxStatusData/Tx Sec Status ID120/Float Data to Bytes ==
  Float Data : Inport
  Resol. : Inport  Port=2
  Bit Shift : hdlsllib/Logic and Bit Operations/Bit Shift  mode=Shift Right Logical  N=8
  Bitwise AND : simulink/Logic and Bit Operations/Bitwise Operator  logicop=AND  UseBitMask=on  BitMask=bin2dec('0000000011111111')  BitMaskRealWorld=Stored Integer
  Bitwise AND1 : simulink/Logic and Bit Operations/Bitwise Operator  logicop=AND  UseBitMask=on  BitMask=hex2dec('FF00')  BitMaskRealWorld=Stored Integer
  Data Type Conversion : DataTypeConversion  OutDataTypeStr=uint8  SaturateOnIntegerOverflow=off  RndMeth=Floor
  Data Type Conversion1 : DataTypeConversion  OutDataTypeStr=uint8  SaturateOnIntegerOverflow=off  RndMeth=Floor
  Data Type Conversion2 : DataTypeConversion  OutDataTypeStr=uint16  SaturateOnIntegerOverflow=off  RndMeth=Floor
  Divide : Product  Inputs=*/
  u8Lsb : Outport
  u8Msb : Outport  Port=2
  wires:
  Data Type Conversion/1 -> u8Lsb/1
  Bitwise AND1/1 -> Bit Shift/1
  Data Type Conversion1/1 -> u8Msb/1
  Bitwise AND/1 -> Data Type Conversion/1
  Bit Shift/1 -> Data Type Conversion1/1
  Data Type Conversion2/1 -> Bitwise AND1/1, Bitwise AND/1  "u16toBytes_1"
  Divide/1 -> Data Type Conversion2/1
  Float Data/1 -> Divide/1
  Resol./1 -> Divide/2

== system main/Task_Manager/Tmr_20mS/codegen/Task_20mS/Tx_Handler/Run Tx Routine/TxStatusData/Tx Sec Status ID120/Float Data to Bytes1 ==
  Float Data : Inport
  Resol. : Inport  Port=2
  Bit Shift : hdlsllib/Logic and Bit Operations/Bit Shift  mode=Shift Right Logical  N=8
  Bitwise AND : simulink/Logic and Bit Operations/Bitwise Operator  logicop=AND  UseBitMask=on  BitMask=bin2dec('0000000011111111')  BitMaskRealWorld=Stored Integer
  Bitwise AND1 : simulink/Logic and Bit Operations/Bitwise Operator  logicop=AND  UseBitMask=on  BitMask=hex2dec('FF00')  BitMaskRealWorld=Stored Integer
  Data Type Conversion : DataTypeConversion  OutDataTypeStr=uint8  SaturateOnIntegerOverflow=off  RndMeth=Floor
  Data Type Conversion1 : DataTypeConversion  OutDataTypeStr=uint8  SaturateOnIntegerOverflow=off  RndMeth=Floor
  Data Type Conversion2 : DataTypeConversion  OutDataTypeStr=uint16  SaturateOnIntegerOverflow=off  RndMeth=Floor
  Divide : Product  Inputs=*/
  u8Lsb : Outport
  u8Msb : Outport  Port=2
  wires:
  Resol./1 -> Divide/2
  Float Data/1 -> Divide/1
  Divide/1 -> Data Type Conversion2/1
  Data Type Conversion2/1 -> Bitwise AND/1, Bitwise AND1/1  "u16toBytes_1"
  Bit Shift/1 -> Data Type Conversion1/1
  Bitwise AND/1 -> Data Type Conversion/1
  Data Type Conversion1/1 -> u8Msb/1
  Bitwise AND1/1 -> Bit Shift/1
  Data Type Conversion/1 -> u8Lsb/1

== system main/Task_Manager/Tmr_20mS/codegen/Task_20mS/Tx_Handler/Run Tx Routine/TxStatusData/Tx Sec Status ID120/Float Data to Bytes2 ==
  Float Data : Inport
  Resol. : Inport  Port=2
  Bit Shift : hdlsllib/Logic and Bit Operations/Bit Shift  mode=Shift Right Logical  N=8
  Bitwise AND : simulink/Logic and Bit Operations/Bitwise Operator  logicop=AND  UseBitMask=on  BitMask=bin2dec('0000000011111111')  BitMaskRealWorld=Stored Integer
  Bitwise AND1 : simulink/Logic and Bit Operations/Bitwise Operator  logicop=AND  UseBitMask=on  BitMask=hex2dec('FF00')  BitMaskRealWorld=Stored Integer
  Data Type Conversion : DataTypeConversion  OutDataTypeStr=uint8  SaturateOnIntegerOverflow=off  RndMeth=Floor
  Data Type Conversion1 : DataTypeConversion  OutDataTypeStr=uint8  SaturateOnIntegerOverflow=off  RndMeth=Floor
  Data Type Conversion2 : DataTypeConversion  OutDataTypeStr=uint16  SaturateOnIntegerOverflow=off  RndMeth=Floor
  Divide : Product  Inputs=*/
  u8Lsb : Outport
  u8Msb : Outport  Port=2
  wires:
  Data Type Conversion/1 -> u8Lsb/1
  Bitwise AND1/1 -> Bit Shift/1
  Data Type Conversion1/1 -> u8Msb/1
  Bitwise AND/1 -> Data Type Conversion/1
  Bit Shift/1 -> Data Type Conversion1/1
  Data Type Conversion2/1 -> Bitwise AND1/1, Bitwise AND/1  "u16toBytes_1"
  Divide/1 -> Data Type Conversion2/1
  Float Data/1 -> Divide/1
  Resol./1 -> Divide/2

== system main/Task_Manager/Tmr_20mS/codegen/Task_20mS/Tx_Handler/Run Tx Routine/TxStatusData/Tx Sec Status ID120/TxReadRequest ==
  Action Port : ActionPort  ActionPortLabel=if(u1 == 1 )
  Constant1 : Constant  OutDataTypeStr=uint8
  Data Store Write1 : DataStoreWrite  DataStoreName=u8CanTxIndex  IndexOptions=Index vector (dialog)  Indices=1  OutputSizes=1
  wires:
  Constant1/1 -> Data Store Write1/1

== system main/Task_Manager/Tmr_20mS/codegen/Task_20mS/Tx_Handler/Run Tx Routine/TxStatusData/Tx Sec Status ID120/u16 Data to Bytes ==
  u16 Data : Inport
  Bit Shift : hdlsllib/Logic and Bit Operations/Bit Shift  mode=Shift Right Logical  N=8
  Bitwise AND : simulink/Logic and Bit Operations/Bitwise Operator  logicop=AND  UseBitMask=on  BitMask=bin2dec('0000000011111111')  BitMaskRealWorld=Stored Integer
  Bitwise AND1 : simulink/Logic and Bit Operations/Bitwise Operator  logicop=AND  UseBitMask=on  BitMask=hex2dec('FF00')  BitMaskRealWorld=Stored Integer
  Data Type Conversion : DataTypeConversion  OutDataTypeStr=uint8  SaturateOnIntegerOverflow=off  RndMeth=Floor
  Data Type Conversion1 : DataTypeConversion  OutDataTypeStr=uint8  SaturateOnIntegerOverflow=off  RndMeth=Floor
  u8Lsb : Outport
  u8Msb : Outport  Port=2
  wires:
  u16 Data/1 -> Bitwise AND1/1, Bitwise AND/1
  Bit Shift/1 -> Data Type Conversion1/1
  Bitwise AND/1 -> Data Type Conversion/1
  Data Type Conversion1/1 -> u8Msb/1
  Bitwise AND1/1 -> Bit Shift/1
  Data Type Conversion/1 -> u8Lsb/1

== system main/Task_Manager/Tmr_20mS/codegen/Task_20mS/Tx_Handler/Run Tx Routine/TxStatusData/Tx Sec1 ID140/Float Data to Bytes2 ==
  Float Data : Inport
  Resol. : Inport  Port=2
  Bit Shift : hdlsllib/Logic and Bit Operations/Bit Shift  mode=Shift Right Logical  N=8
  Bitwise AND : simulink/Logic and Bit Operations/Bitwise Operator  logicop=AND  UseBitMask=on  BitMask=bin2dec('0000000011111111')  BitMaskRealWorld=Stored Integer
  Bitwise AND1 : simulink/Logic and Bit Operations/Bitwise Operator  logicop=AND  UseBitMask=on  BitMask=hex2dec('FF00')  BitMaskRealWorld=Stored Integer
  Data Type Conversion : DataTypeConversion  OutDataTypeStr=uint8  SaturateOnIntegerOverflow=off  RndMeth=Floor
  Data Type Conversion1 : DataTypeConversion  OutDataTypeStr=uint8  SaturateOnIntegerOverflow=off  RndMeth=Floor
  Data Type Conversion2 : DataTypeConversion  OutDataTypeStr=uint16  SaturateOnIntegerOverflow=off  RndMeth=Floor
  Divide : Product  Inputs=*/
  u8Lsb : Outport
  u8Msb : Outport  Port=2
  wires:
  Data Type Conversion/1 -> u8Lsb/1
  Bitwise AND1/1 -> Bit Shift/1
  Data Type Conversion1/1 -> u8Msb/1
  Bitwise AND/1 -> Data Type Conversion/1
  Bit Shift/1 -> Data Type Conversion1/1
  Data Type Conversion2/1 -> Bitwise AND1/1, Bitwise AND/1  "u16toBytes_1"
  Divide/1 -> Data Type Conversion2/1
  Float Data/1 -> Divide/1
  Resol./1 -> Divide/2

== system main/Task_Manager/Tmr_20mS/codegen/Task_20mS/Tx_Handler/Run Tx Routine/TxStatusData/Tx Sec1 ID140/u16 Data to Bytes ==
  u16 Data : Inport
  Bit Shift : hdlsllib/Logic and Bit Operations/Bit Shift  mode=Shift Right Logical  N=8
  Bitwise AND : simulink/Logic and Bit Operations/Bitwise Operator  logicop=AND  UseBitMask=on  BitMask=bin2dec('0000000011111111')  BitMaskRealWorld=Stored Integer
  Bitwise AND1 : simulink/Logic and Bit Operations/Bitwise Operator  logicop=AND  UseBitMask=on  BitMask=hex2dec('FF00')  BitMaskRealWorld=Stored Integer
  Data Type Conversion : DataTypeConversion  OutDataTypeStr=uint8  SaturateOnIntegerOverflow=off  RndMeth=Floor
  Data Type Conversion1 : DataTypeConversion  OutDataTypeStr=uint8  SaturateOnIntegerOverflow=off  RndMeth=Floor
  u8Lsb : Outport
  u8Msb : Outport  Port=2
  wires:
  u16 Data/1 -> Bitwise AND1/1, Bitwise AND/1
  Bit Shift/1 -> Data Type Conversion1/1
  Bitwise AND/1 -> Data Type Conversion/1
  Data Type Conversion1/1 -> u8Msb/1
  Bitwise AND1/1 -> Bit Shift/1
  Data Type Conversion/1 -> u8Lsb/1

== system main/Task_Manager/Tmr_20mS/codegen/Task_20mS/Tx_Handler/Run Tx Routine/TxStatusData/Tx Sec1 ID140/u16 Data to Bytes1 ==
  u16 Data : Inport
  Bit Shift : hdlsllib/Logic and Bit Operations/Bit Shift  mode=Shift Right Logical  N=8
  Bitwise AND : simulink/Logic and Bit Operations/Bitwise Operator  logicop=AND  UseBitMask=on  BitMask=bin2dec('0000000011111111')  BitMaskRealWorld=Stored Integer
  Bitwise AND1 : simulink/Logic and Bit Operations/Bitwise Operator  logicop=AND  UseBitMask=on  BitMask=hex2dec('FF00')  BitMaskRealWorld=Stored Integer
  Data Type Conversion : DataTypeConversion  OutDataTypeStr=uint8  SaturateOnIntegerOverflow=off  RndMeth=Floor
  Data Type Conversion1 : DataTypeConversion  OutDataTypeStr=uint8  SaturateOnIntegerOverflow=off  RndMeth=Floor
  u8Lsb : Outport
  u8Msb : Outport  Port=2
  wires:
  Data Type Conversion/1 -> u8Lsb/1
  Bitwise AND1/1 -> Bit Shift/1
  Data Type Conversion1/1 -> u8Msb/1
  Bitwise AND/1 -> Data Type Conversion/1
  Bit Shift/1 -> Data Type Conversion1/1
  u16 Data/1 -> Bitwise AND/1, Bitwise AND1/1
